simulink model "EcoSIM3_P2_C2_WIP"  (R2014b)
settings: Solver=ode1  SolverMode=SingleTasking  StartTime=0.0  StopTime=inf  FixedStep=0.01  RelTol=1e-3
PostLoadFcn:
  | %, if any(exist('dsrtsu_mdlpostloadfcn', 'file') == [2, 3, 6]), try dsrtsu_mdlpostloadfcn('Execute', bdroot); catch fprintf('Error in PostLoadFcn (dsrtsu_mdlpostloadfcn) for model "%s":\n %s\n', bdroot, lasterr); end, end,
InitFcn:
  | tic
  | %Startup_EcoSIM
values from neighbouring files (symbols this model uses):
  EngPwr = [0 5	10	15	20	25	30	35	40	45	50	55	60	65	70	75	80	85	90	95	100	105	110	115]    [Series_Maps.m]
  EngSpd = [0 477.4645 954.929 1909.858 2864.787 3819.716 4774.645 5729.574 6684.503]    [Series_Maps.m]
  EngTrq = [0	0	0	0	0	0	0	0	0	0	0	0	0	0	0	0	0	0	0	0	0	0	0	0 ... (first row only)    [Series_Maps.m]
  Power = [0 5 10 15 20 25 30]    [Series_Maps.m]
  Torque = [-50,-40,-30,-25,-20,-15,-10,-8,-6,-4,-2,0]    [Series_Maps.m]
undefined symbols (not defined in the file or in its folder): canChannel, Controls, DriveCycles, Driver, EM_EFF_MAP, EM_PwrLoss_MAP, Glbl, Overwritten_Mode, Plants, sigbuilder_block, Trialmap, Veh_Dynamics
libraries: simulink x141, canmsglib x113, fl_lib x104, canlib x89, nesl_utility x56, sdl_lib x29, dspsigops x6, dspswit3 x5, dspstat3 x2, commnoisgen2 x1, dspfdesign x1
(part 4 of 21)

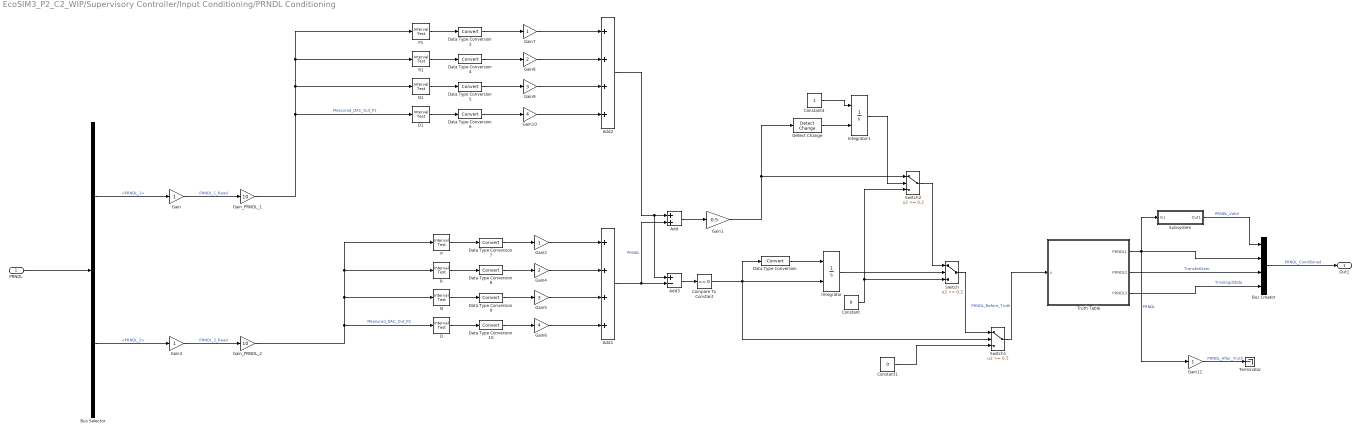
== system EcoSIM3_P2_C2_WIP/Supervisory Controller/Input Conditioning/PRNDL Conditioning ==
  PRNDL : Inport
  Add : Sum
  Add1 : Sum  Inputs=++++
  Add2 : Sum  Inputs=++++
  Add3 : Sum  Inputs=+-
  Bus Creator : BusCreator
  Bus Selector : BusSelector  OutputSignals=GM_Transmit.GM_Electrical_Out.PRNDL_1,GM_Transmit.GM_Electrical_Out.PRNDL_2
  Compare To Constant : simulink/Logic and Bit Operations/Compare To Constant  relop===  const=0  OutDataTypeStr=boolean
  Constant : Constant  Value=0
  Constant1 : Constant  Value=0
  Constant4 : Constant
  D : simulink/Logic and Bit Operations/Interval Test  IntervalClosedRight=on  uplimit=1.90  IntervalClosedLeft=on  lowlimit=1.70  OutDataTypeStr=boolean
  D1 : simulink/Logic and Bit Operations/Interval Test  IntervalClosedRight=on  uplimit=2.2  IntervalClosedLeft=on  lowlimit=1.9  OutDataTypeStr=boolean
  Data Type Conversion{,3..10} (9 alike) : DataTypeConversion
  Detect Change : simulink/Logic and Bit Operations/Detect Change  vinit=0  InputProcessing=Inherited  OutDataTypeStr=boolean
  Gain{,2..3,7,11} (5 alike) : Gain
  Gain1 : Gain  Gain=0.5
  Gain10 : Gain  Gain=4
  Gain4 : Gain  Gain=2
  Gain5 : Gain  Gain=3
  Gain6 : Gain  Gain=4
  Gain8 : Gain  Gain=2
  Gain9 : Gain  Gain=3
  Gain_PRNDL_1 : Gain  Gain=10
  Gain_PRNDL_2 : Gain  Gain=10
  Integrator : Integrator  ExternalReset=either
  Integrator1 : Integrator  ExternalReset=either
  N : simulink/Logic and Bit Operations/Interval Test  IntervalClosedRight=on  uplimit=1.65  IntervalClosedLeft=on  lowlimit=1.35  OutDataTypeStr=boolean
  N1 : simulink/Logic and Bit Operations/Interval Test  IntervalClosedRight=on  uplimit=1.80  IntervalClosedLeft=on  lowlimit=1.55  OutDataTypeStr=boolean
  P : simulink/Logic and Bit Operations/Interval Test  IntervalClosedRight=on  uplimit=0.6  IntervalClosedLeft=on  lowlimit=0.3  OutDataTypeStr=boolean
  P1 : simulink/Logic and Bit Operations/Interval Test  IntervalClosedRight=on  uplimit=0.80  IntervalClosedLeft=on  lowlimit=0.55  OutDataTypeStr=boolean
  R : simulink/Logic and Bit Operations/Interval Test  IntervalClosedRight=on  uplimit=1.25  IntervalClosedLeft=on  lowlimit=1.0  OutDataTypeStr=boolean
  R1 : simulink/Logic and Bit Operations/Interval Test  IntervalClosedRight=on  uplimit=1.45  IntervalClosedLeft=on  lowlimit=1.20  OutDataTypeStr=boolean
  Subsystem : Subsystem
  Switch : Switch  Threshold=0.2
  Switch1 : Switch  Threshold=0.5
  Switch2 : Switch  Threshold=0.2
  Terminator : Terminator
  Truth Table : Truth Table  TreatAsAtomicUnit=on
  Out1 : Outport
  wires:
  Gain_PRNDL_2/1 -> R/1, P/1, N/1, D/1  "Measured_DAC_Out_P2"
  Gain3/1 -> Gain_PRNDL_2/1  "PRNDL_2_Read"
  Bus Selector/2 -> Gain3/1  "<PRNDL_2>"
  Gain_PRNDL_1/1 -> D1/1, N1/1, R1/1, P1/1  "Measured_DAC_Out_P1"
  Gain/1 -> Gain_PRNDL_1/1  "PRNDL_1_Read"
  Bus Selector/1 -> Gain/1  "<PRNDL_1>"
  PRNDL/1 -> Bus Selector/1
  Data Type Conversion7/1 -> Gain2/1
  Data Type Conversion8/1 -> Gain4/1
  Data Type Conversion10/1 -> Gain6/1
  Gain2/1 -> Add1/1
  Gain4/1 -> Add1/2
  Gain5/1 -> Add1/3
  Gain6/1 -> Add1/4
  Data Type Conversion9/1 -> Gain5/1
  Truth Table/1(PRNDL1) -> Bus Creator/2, Subsystem/1(In1), Gain11/1  "PRNDL"
  Truth Table/2(PRNDL2) -> Bus Creator/3  "TransEstGear"
  Truth Table/3(PRNDL3) -> Bus Creator/4  "TrnsEngdState"
  Subsystem/1(Out1) -> Bus Creator/1  "PRNDL_Valid"
  Bus Creator/1 -> Out1/1  "PRNDL_Conditioned"
  P1/1 -> Data Type Conversion3/1
  R1/1 -> Data Type Conversion4/1
  D1/1 -> Data Type Conversion6/1
  Gain7/1 -> Add2/1
  Gain8/1 -> Add2/2
  Gain9/1 -> Add2/3
  Gain10/1 -> Add2/4
  N1/1 -> Data Type Conversion5/1
  Add2/1 -> Add3/1, Add/1
  Add1/1 -> Add/2, Add3/2  "PRNDL"
  Add/1 -> Gain1/1
  Add3/1 -> Compare To Constant/1
  Data Type Conversion/1 -> Integrator/1
  Integrator/1 -> Switch/2
  Constant/1 -> Switch2/3, Switch/3
  Switch1/1 -> Truth Table/1(u)  "PRNDL_Before_Truth"
  Data Type Conversion6/1 -> Gain10/1
  Data Type Conversion5/1 -> Gain9/1
  Data Type Conversion4/1 -> Gain8/1
  Data Type Conversion3/1 -> Gain7/1
  P/1 -> Data Type Conversion7/1
  R/1 -> Data Type Conversion8/1
  D/1 -> Data Type Conversion10/1
  N/1 -> Data Type Conversion9/1
  Compare To Constant/1 -> Integrator/2, Switch1/2, Data Type Conversion/1
  Switch/1 -> Switch1/1
  Constant1/1 -> Switch1/3
  Detect Change/1 -> Integrator1/2
  Constant4/1 -> Integrator1/1
  Integrator1/1 -> Switch2/2
  Gain1/1 -> Detect Change/1, Switch2/1
  Switch2/1 -> Switch/1
  Gain11/1 -> Terminator/1  "PRNDL_After_Truth"

== system EcoSIM3_P2_C2_WIP/Supervisory Controller/Input Conditioning/Velocity Conditioning ==
  Raw Ticks : Inport
  Bus Creator : BusCreator  Inputs=2
  Bus Selector1 : BusSelector  OutputSignals=GM_Transmit.GMLAN_CAN_Out.PPEI_Vehicle_Speed_and_Distance.VehSpdAvgDrvn,GM_Transmit.GMLAN_CAN_Out.PPEI_Driven_Whl_Rotational_Stat.WRSLDWhlDistPlsCntr,GM_Transmit.GMLAN_CAN_Out.PPEI_Driven_Whl_Rotational_Stat.WRSRDWhlDistPlsCntr,GM_Transmit.GMLAN_CAN_Out.PPEI_NonDrivn_Whl_Rotationl_Stat.WRSLNDWhlDistPCntr,GM_Transmit.GMLAN_CAN_Out.PPEI_NonDrivn_Whl_Rotationl_Stat.WRSRNDWhlDistPCntr
  Gain : Gain  Gain=1/3.6
  Mean : dspstat3/Mean  run=off  reset_popup=None  InputProcessing=Columns as channels (frame based)  directionMode=Each column  dimension=1  treatSBRowAsCol=on  roiEnable=off  roiType=Rectangles  roiPortion=Entire ROI  roiOutput=Individual statistics for each ROI  roiFlag=off  outputDataTypeStr=Inherit: Same as accumulator  outputLastDataTypeStr=Inherit: Same as accumulator  outputMin=[]  outputMax=[]  roundingMode=Floor  overflowMode=off
  Mux : Mux
  Subsystem : Subsystem
  Subsystem1 : Subsystem
  Subsystem2 : Subsystem
  Subsystem3 : Subsystem
  Velocity Processed : Outport
  wires:
  Bus Selector1/5 -> Subsystem3/1(In1)  "<WRSRNDWhlDistPCntr>"
  Bus Selector1/4 -> Subsystem2/1(In1)  "<WRSLNDWhlDistPCntr>"
  Raw Ticks/1 -> Bus Selector1/1
  Bus Selector1/1 -> Gain/1  "<VehSpdAvgDrvn>"
  Bus Selector1/3 -> Subsystem1/1(In1)  "<WRSRDWhlDistPlsCntr>"
  Bus Creator/1 -> Velocity Processed/1  "Vehicle_speed"
  Mean/1 -> Bus Creator/2  "Processed_Speed_m_per_sec"
  Gain/1 -> Bus Creator/1  "Vehicle_Speed_meter_per_s"
  Bus Selector1/2 -> Subsystem/1(In1)  "<WRSLDWhlDistPlsCntr>"
  Subsystem2/1(Speed_LND) -> Mux/3
  Subsystem1/1(Speed_RD) -> Mux/2
  Subsystem/1(Speed_LD) -> Mux/1
  Subsystem3/1(Speed_RND) -> Mux/4
  Mux/1 -> Mean/1

== system EcoSIM3_P2_C2_WIP/Supervisory Controller/Mode Operation/Accessory ==
  "Supervisory " : Inport
  CAN : Inport  Port=2
  Enable : EnablePort  StatesWhenEnabling=reset
  BAS_Signals : Subsystem  Commented=on
  BAS_Signals1 : Subsystem
  Bus Creator2 : BusCreator  Inputs=8
  Constant1 : Constant  Value=0
  DC/DC Enabled : Subsystem
  ESS_Messages : Subsystem
  Engine Messages : Subsystem
  Signal Conversion : SignalConversion
  TM Messages : Subsystem
  Trans_Messages : Subsystem
  Output : Outport
  wires:
  Signal Conversion/1 -> Output/1  "HSC_Output"
  Engine Messages/1(Out1) -> Bus Creator2/5
  ESS_Messages/1(Out1) -> Bus Creator2/2  "ESS_Signals_A123"
  Trans_Messages/1(Out1) -> Bus Creator2/6  "Trans_Receive"
  "Supervisory "/1 -> Bus Creator2/7  "Supervisory"
  Bus Creator2/1 -> Signal Conversion/1  "HSC_Output"
  DC/DC Enabled/1(Out1) -> Bus Creator2/8
  TM Messages/1(Out1) -> Bus Creator2/3
  Constant1/1 -> Bus Creator2/1  "Vehicle_Ready"
  CAN/1 -> BAS_Signals1/1(BAS_Speed)
  BAS_Signals1/1(Signals) -> Bus Creator2/4

== system EcoSIM3_P2_C2_WIP/Supervisory Controller/Mode Operation/Charging ==
  From CAN : Inport
  "Supervisory " : Inport  Port=2
  Enable : EnablePort  StatesWhenEnabling=reset
  BAS_Signals : Subsystem  Commented=on
  BAS_Signals1 : Subsystem
  Bus Creator2 : BusCreator  Inputs=8
  Constant2 : Constant  Value=0
  DC/DC Enabled : Subsystem
  EM_Signals : Subsystem
  ESS_Messages : Subsystem
  Engine Messages : Subsystem
  Signal Conversion : SignalConversion
  Trans_Messages : Subsystem
  Output : Outport
  wires:
  Signal Conversion/1 -> Output/1  "HSC_Output"
  Engine Messages/1(Out1) -> Bus Creator2/5
  ESS_Messages/1(Out1) -> Bus Creator2/2  "ESS_Signals_A123"
  Trans_Messages/1(Out1) -> Bus Creator2/6  "Trans_Receive"
  From CAN/1 -> BAS_Signals1/1(BAS_Speed), ESS_Messages/1(From CAN)
  "Supervisory "/1 -> Bus Creator2/7  "Supervisory"
  Bus Creator2/1 -> Signal Conversion/1  "HSC_Output"
  EM_Signals/1(Out1) -> Bus Creator2/3
  DC/DC Enabled/1(Out1) -> Bus Creator2/8
  Constant2/1 -> Bus Creator2/1  "Vehicle_Ready"
  BAS_Signals1/1(Signals) -> Bus Creator2/4

== system EcoSIM3_P2_C2_WIP/Supervisory Controller/Mode Operation/EV ==
  "Supervisory " : Inport
  CAN : Inport  Port=2
  Enable : EnablePort  StatesWhenEnabling=reset
  BAS_Signals : Subsystem  Commented=on
  BAS_Signals1 : Subsystem
  Bus Creator1 : BusCreator  Inputs=8
  Bus Creator2 : BusCreator  Inputs=3
  Bus Selector : BusSelector  OutputSignals=Driver Torque Request
  Bus Selector1 : BusSelector  OutputSignals=EM_Transmit.EM_CAN_Out.M165_Motor_Position_Info.Motor_Speed,EM_Transmit.EM_CAN_Out.M162_Temperature_Set_3.Motor_Temperature
  Constant1 : Constant  Value=0
  Constant2 : Constant
  Constant4 : Constant
  Constant5 : Constant  Value=0
  DC/DC Enabled : Subsystem
  EM Max Torque1 : Lookup_n-D  NumberOfTableDimensions=1  BreakpointsForDimension1=Plants.EM.Mdl.Plant.max_min_RPM  BreakpointsForDimension2=[25,70]  Table=[Plants.EM.Mdl.Plant.T_max_Peak]  InternalRulePriority=Speed  RndMeth=Simplest  InputSameDT=on
  ESS_Messages : Subsystem
  Engine Messages : Subsystem
  Gain : Gain  Gain=1/(2.77*2.77)
  Saturation Dynamic : simulink/Discontinuities/Saturation Dynamic  OutMin=[]  OutMax=[]  OutDataTypeStr=Inherit: Same as second input  OutDataType=fixdt(1, 16)  OutScaling=2^-10  DoSatur=off
  Scope : Scope
      settings: SaveName=ScopeData67
  Signal Conversion : SignalConversion
  Trans_Messages : Subsystem
  Output : Outport
  wires:
  Signal Conversion/1 -> Output/1  "HSC_Output"
  Engine Messages/1(Out1) -> Bus Creator1/5
  ESS_Messages/1(Out1) -> Bus Creator1/2  "ESS_Signals_A123"
  Bus Creator2/1 -> Bus Creator1/3  "EM_Messages_Rhinehart"
  Gain/1 -> Saturation Dynamic/2  "Torque_Command"
  Constant1/1 -> Bus Creator2/3  "Rotation_Direction"
  Constant2/1 -> Bus Creator2/1  "Inverter_Enable"
  Trans_Messages/1(Out1) -> Bus Creator1/6  "Trans_Receive"
  "Supervisory "/1 -> Bus Creator1/7, Bus Selector/1  "Supervisory"
  Bus Creator1/1 -> Signal Conversion/1  "HSC_Output"
  Bus Selector/1 -> Gain/1  "<Driver Torque Request>"
  Constant4/1 -> Bus Creator1/1  "Vehicle_Ready"
  DC/DC Enabled/1(Out1) -> Bus Creator1/8
  Saturation Dynamic/1 -> Bus Creator2/2  "Torque_Command"
  Constant5/1 -> Saturation Dynamic/3
  CAN/1 -> BAS_Signals1/1(BAS_Speed), Bus Selector1/1
  Bus Selector1/1 -> EM Max Torque1/1  "<Motor_Speed>"
  Bus Selector1/2 -> ?  "<Motor_Temperature>"
  EM Max Torque1/1 -> Scope/1, Saturation Dynamic/1
  BAS_Signals1/1(Signals) -> Bus Creator1/4

== system EcoSIM3_P2_C2_WIP/Supervisory Controller/Mode Operation/Engine Only  ==
  note: this will end up being engine idle in the vehicle
  "Supervisory " : Inport
  From CAN : Inport  Port=2
  Enable : EnablePort  StatesWhenEnabling=reset
  BAS_Signals : Subsystem  Commented=on
  BAS_Signals1 : Subsystem
  Bus Creator1 : BusCreator  Inputs=8
  Bus Creator6 : BusCreator  Commented=on  Inputs=2
  Constant1 : Constant  Commented=on
  Constant2 : Constant  Commented=on  Value=0
  Constant4 : Constant
  DC/DC Enabled : Subsystem
  ESS_Messages : Subsystem
  Engine Messages : Subsystem  Commented=on
  Engine Messages1 : Subsystem
  "ICE Torque Request & Gear Selection " : Subsystem
  Signal Conversion : SignalConversion
  Subsystem : Subsystem  Commented=on
  Supervisory 1 : InportShadow
  TM Messages : Subsystem
  Terminator : Terminator  Commented=on
  Terminator1 : Terminator  Commented=on
  Trans Clutch Messages : Subsystem
  "Output " : Outport
  wires:
  Signal Conversion/1 -> "Output "/1  "HSC_Output"
  ESS_Messages/1(Out1) -> Bus Creator1/2  "ESS_Signals_A123"
  BAS_Signals1/1(Signals) -> Bus Creator1/4
  Subsystem/3("Gear Requested ") -> Terminator1/1  "Gear_Request"
  "Supervisory "/1 -> Bus Creator1/7  "Supervisory"
  Bus Creator1/1 -> Signal Conversion/1  "HSC_Output"
  Subsystem/2(Shift Requested) -> Terminator/1
  Constant4/1 -> Bus Creator1/1  "Vehicle_Ready"
  DC/DC Enabled/1(Out1) -> Bus Creator1/8
  TM Messages/1(Out1) -> Bus Creator1/3  "EM_Messages_Rhinehart"
  Engine Messages1/1(Out1) -> Bus Creator1/5
  Supervisory 1/1 -> TM Messages/1(Supervisory)  "Supervisory"
  From CAN/1 -> "ICE Torque Request & Gear Selection "/1(CAN), Trans Clutch Messages/2(CAN), TM Messages/2(CAN), BAS_Signals1/1(BAS_Speed)
  "ICE Torque Request & Gear Selection "/1(ICE_Torque_Request [Nm]) -> Engine Messages1/1(Torque)
  "ICE Torque Request & Gear Selection "/2(Gear_Request[-]) -> Trans Clutch Messages/1(Gear Request)
  Trans Clutch Messages/1(Out1) -> Bus Creator1/6
  Constant2/1 -> Bus Creator6/1  "Shift_Request"
  Constant1/1 -> Bus Creator6/2  "Gear_Request"

== system EcoSIM3_P2_C2_WIP/Supervisory Controller/Mode Operation/Engine Start  ==
  "Supervisory " : Inport
  "CAN In " : Inport  Port=2
  Enable : EnablePort  StatesWhenEnabling=reset
  1-D Lookup Table : Lookup_n-D  NumberOfTableDimensions=1  BreakpointsForDimension1=[0 2699 2700 3000 3239 3240]  Table=[11.11 11.11 8 5.5 5.5 0]  InternalRulePriority=Speed  RndMeth=Simplest  InputSameDT=on
  BAS_Signals1 : Subsystem
  Bus Creator1 : BusCreator  Inputs=8
  Bus Creator2 : BusCreator  Inputs=3
  Bus Creator4 : BusCreator  Inputs=3
  Bus Selector : BusSelector  OutputSignals=BAS_Transmit.BAS_CAN_Out.Status_1.BAS_Speed_rad_per_s
  Compare To Constant : simulink/Logic and Bit Operations/Compare To Constant  relop=>  const=900  OutDataTypeStr=boolean
  Constant1 : Constant  Value=0
  Constant3 : Constant  Value=0
  Constant4 : Constant
  Constant5 : Constant
  Constant6 : Constant
  Convert to Engine Speed : Gain  Gain=1/2.7
  DC/DC Enabled : Subsystem
  Data Type Conversion : DataTypeConversion  OutDataTypeStr=double
  ESS_Messages : Subsystem
  Engine Messages : Subsystem
  Sample and Hold : dspsigops/Sample and Hold  trig=Rising edge  initCond=0  latchinput=off
  Signal Conversion : SignalConversion
  Supervisory 1 : InportShadow
  TM Messages : Subsystem
  Trans Messages : Subsystem
  rad/sec to RPM : Gain  Gain=9.54929659643
  rad/sec to RPM1 : Gain  Gain=1.1
  "Output " : Outport
  wires:
  Signal Conversion/1 -> "Output "/1  "HSC_Output"
  ESS_Messages/1(Out1) -> Bus Creator1/2  "ESS_Signals_A123"
  "Supervisory "/1 -> Bus Creator1/7  "Supervisory"
  Bus Creator1/1 -> Signal Conversion/1  "HSC_Output"
  Constant5/1 -> Bus Creator1/1  "Vehicle_Ready"
  DC/DC Enabled/1(Out1) -> Bus Creator1/8
  TM Messages/1(Out1) -> Bus Creator1/3
  Constant6/1 -> Bus Creator4/3  "BAS_Mode_Request"
  Trans Messages/1(Out1) -> Bus Creator1/6
  Supervisory 1/1 -> TM Messages/1(In1)  "Supervisory"
  Constant3/1 -> Bus Creator2/1  "ICE_Torque_Request_Nm"
  1-D Lookup Table/1 -> rad/sec to RPM1/1  "BAS_Torque_Request_Nm"
  Constant1/1 -> Bus Creator4/2  "BAS_Speed_Request"
  Constant4/1 -> Bus Creator2/2  "Engine_On"
  "CAN In "/1 -> BAS_Signals1/1(BAS_Speed), Bus Selector/1
  Bus Selector/1 -> Engine Messages/1(In1), rad/sec to RPM/1  "<BAS_Speed_rad_per_s>"
  rad/sec to RPM/1 -> 1-D Lookup Table/1, Convert to Engine Speed/1  "BAS_Speed_RPM"
  Compare To Constant/1 -> Data Type Conversion/1
  Convert to Engine Speed/1 -> Compare To Constant/1
  Data Type Conversion/1 -> Sample and Hold/Trigger, Sample and Hold/1  "Engine_Run"
  Sample and Hold/1 -> Bus Creator2/3  "Engine_Run"
  rad/sec to RPM1/1 -> Bus Creator4/1  "BAS_Torque_Request_Nm"
  BAS_Signals1/1(Signals) -> Bus Creator1/4
  Engine Messages/1(Out1) -> Bus Creator1/5

== system EcoSIM3_P2_C2_WIP/Supervisory Controller/Mode Operation/Limited EV ==
  "Supervisory " : Inport
  CAN : Inport  Port=2
  Enable : EnablePort  StatesWhenEnabling=reset
  BAS_Signals : Subsystem  Commented=on
  BAS_Signals1 : Subsystem
  Bus Creator3 : BusCreator  Inputs=8
  Bus Creator4 : BusCreator  Inputs=3
  Bus Selector : BusSelector  OutputSignals=Driver Torque Request
  Bus Selector1 : BusSelector  OutputSignals=ESS_Transmit.ESS_CAN_Out.BCM_Limits.bcm_dis_buf,EM_Transmit.EM_CAN_Out.M162_Temperature_Set_3.Motor_Temperature,EM_Transmit
  Constant1 : Constant
  Constant2 : Constant  Value=0
  Constant4 : Constant
  DC/DC Enabled : Subsystem
  ESS_Messages : Subsystem
  Gain1 : Gain  Gain=1/(2.77*2.77)
  ICE_torque : Subsystem
  "Inverter Temp Selection " : Subsystem
  Signal Conversion : SignalConversion
  Subsystem : Subsystem
  Temperature Limiting Disbuf : Subsystem
  Temperature Limiting Old : Subsystem  Commented=on
  Output : Outport
  wires:
  Signal Conversion/1 -> Output/1  "HSC_Output"
  ESS_Messages/1(Out1) -> Bus Creator3/2  "ESS_Signals_A123"
  Bus Creator4/1 -> Bus Creator3/3  "EM_Messages_Rhinehart"
  Bus Selector/1 -> Subsystem/1(Driver_request), Gain1/1  "<Driver Torque Request>"
  Constant2/1 -> Bus Creator4/3  "Rotation_Direction"
  Constant4/1 -> Bus Creator4/1  "Inverter_Enable"
  "Supervisory "/1 -> Bus Creator3/7, Bus Selector/1  "Supervisory"
  Bus Creator3/1 -> Signal Conversion/1  "HSC_Output"
  Constant1/1 -> Bus Creator3/1  "Vehicle_Ready"
  DC/DC Enabled/1(Out1) -> Bus Creator3/8
  Gain1/1 -> Temperature Limiting Disbuf/2(Torque Request)  "Torque_Command"
  "Inverter Temp Selection "/1(Out1) -> Temperature Limiting Disbuf/5("Inverter Temperature ")
  CAN/1 -> ICE_torque/2(CAN), BAS_Signals1/1(BAS_Speed), Bus Selector1/1
  Temperature Limiting Disbuf/1(EM_torque Command) -> Bus Creator4/2  "Torque_Command"
  Bus Selector1/3 -> "Inverter Temp Selection "/1(In1)  "<EM_Transmit>"
  BAS_Signals1/1(Signals) -> Bus Creator3/4
  Subsystem/1(EM_trq) -> [EM_trq]
  Subsystem/2(ICE_trq) -> [ICE_trq_req]
  [EM_trq] -> Temperature Limiting Disbuf/1(ESS_trq_limit)
  Bus Selector1/2 -> Temperature Limiting Disbuf/4("Motor Temperature ")  "<Motor_Temperature>"
  Bus Selector1/1 -> Subsystem/2(ESS discharge buffer), Temperature Limiting Disbuf/3(ESS discharge buffer)  "<bcm_dis_buf>"
  ICE_torque/2(Trans_Receive) -> Bus Creator3/6
  ICE_torque/1(ICE_Request) -> Bus Creator3/5
  [ICE_trq_req] -> ICE_torque/1(ICE_torque_request)

== system EcoSIM3_P2_C2_WIP/Supervisory Controller/Mode Operation/Series ==
  "Supervisory " : Inport
  From CAN : Inport  Port=2
  Enable : EnablePort  StatesWhenEnabling=reset
  Bus Creator1 : BusCreator  Inputs=8
  Bus Creator2 : BusCreator  Inputs=3
  Bus Creator4 : BusCreator  Inputs=3
  Bus Creator5 : BusCreator  Inputs=3
  Bus Selector : BusSelector  OutputSignals=Driver Torque Request
  Constant1 : Constant  Value=2
  Constant{2,5,7..8} (4 alike) : Constant
  Constant3 : Constant  Value=0
  Constant4 : Constant  Value=0
  DC/DC Enabled : Subsystem
  ESS_Messages : Subsystem
  Gain : Gain
  Gain1 : Gain  Gain=1/(2.77*2.77)
  "Series Torque Determination " : Subsystem
  Signal Conversion : SignalConversion
  Supervisory 1 : InportShadow
  Trans_Messages : Subsystem
  "Output " : Outport
  wires:
  Bus Creator1/1 -> Signal Conversion/1  "HSC_Output"
  "Supervisory "/1 -> Bus Creator1/7  "Supervisory"
  Bus Selector/1 -> Gain1/1  "<Driver Torque Request>"
  Supervisory 1/1 -> Bus Selector/1  "Supervisory"
  Constant5/1 -> Bus Creator5/1  "Inverter_Enable"
  Constant3/1 -> Bus Creator5/3  "Rotation_Direction"
  Bus Creator5/1 -> Bus Creator1/3  "EM_Messages_Rhinehart"
  ESS_Messages/1(Out1) -> Bus Creator1/2  "ESS_Signals_A123"
  Signal Conversion/1 -> "Output "/1  "HSC_Output"
  Trans_Messages/1(Out1) -> Bus Creator1/6  "Trans_Receive"
  Bus Creator4/1 -> Bus Creator1/4  "BAS_SoftECU_Receive"
  Constant1/1 -> Bus Creator4/3  "BAS_Mode_Request"
  DC/DC Enabled/1(Out1) -> Bus Creator1/8
  Constant2/1 -> Bus Creator1/1  "Vehicle_Ready"
  Gain1/1 -> Bus Creator5/2  "Torque_Command"
  "Series Torque Determination "/2(Engine Torque) -> Gain/1
  "Series Torque Determination "/1(BAS Speed) -> Bus Creator4/2  "BAS_Speed_Request"
  Constant4/1 -> Bus Creator4/1  "BAS_Torque_Request_Nm"
  From CAN/1 -> "Series Torque Determination "/1(Battery SOC)
  Gain/1 -> Bus Creator2/1  "ICE_Torque_Request_Nm"
  Constant7/1 -> Bus Creator2/2  "Engine_On"
  Constant8/1 -> Bus Creator2/3  "Engine_Run"
  Bus Creator2/1 -> Bus Creator1/5  "ICE_Request"

== system EcoSIM3_P2_C2_WIP/Supervisory Controller/Mode Operation/Series1 ==
  From CAN : Inport
  "Supervisory " : Inport  Port=2
  Enable : EnablePort  StatesWhenEnabling=reset
  BAS_Signals : Subsystem
  Bus Creator1 : BusCreator  Inputs=8
  Bus Creator2 : BusCreator  Inputs=3
  Bus Selector : BusSelector  OutputSignals=BAS_Transmit.BAS_CAN_Out.Status_1.BAS_Speed_rad_per_s
  Bus Selector1 : BusSelector  OutputSignals=EM_Transmit.EM_CAN_Out.M165_Motor_Position_Info.Motor_Speed
  Bus Selector2 : BusSelector  OutputSignals=Driver Torque Request
  Constant1 : Constant  Value=410
  Constant2 : Constant
  Constant3 : Constant  Value=0
  Constant4 : Constant
  Constant5 : Constant  Value=0
  DC/DC Enabled : Subsystem
  EM Max Torque1 : Lookup_n-D  NumberOfTableDimensions=1  BreakpointsForDimension1=Plants.EM.Mdl.Plant.max_min_RPM  BreakpointsForDimension2=[25,70]  Table=[Plants.EM.Mdl.Plant.T_max_Peak]  InternalRulePriority=Speed  RndMeth=Simplest  InputSameDT=on
  ESS_Messages : Subsystem
  Engine Messages : Subsystem
  Engine Torque Request : Stateflow chart  TreatAsAtomicUnit=on
  Engine Torque Request1 : Stateflow chart  Commented=on  TreatAsAtomicUnit=on
  Gain : Gain  Gain=1/(2.77*2.77)
  Saturation Dynamic : simulink/Discontinuities/Saturation Dynamic  OutMin=[]  OutMax=[]  OutDataTypeStr=Inherit: Same as second input  OutDataType=fixdt(1, 16)  OutScaling=2^-10  DoSatur=off
  Signal Conversion : SignalConversion
  Supervisory 1 : InportShadow  Port=2
  Trans_Messages : Subsystem
  "Output " : Outport
  wires:
  BAS_Signals/1(Signals) -> Bus Creator1/4
  Engine Messages/1(Out1) -> Bus Creator1/5
  DC/DC Enabled/1(Out1) -> Bus Creator1/8
  Constant4/1 -> Bus Creator1/1  "Vehicle_Ready"
  From CAN/1 -> Bus Selector1/1, Bus Selector/1, BAS_Signals/1(BAS_Speed)
  Bus Creator1/1 -> Signal Conversion/1  "HSC_Output"
  "Supervisory "/1 -> Bus Creator1/7  "Supervisory"
  Signal Conversion/1 -> "Output "/1  "HSC_Output"
  Bus Selector/1 -> Engine Torque Request/1(BAS_Speed)  "<BAS_Speed_rad_per_s>"
  Engine Torque Request/1(Torque_Request) -> Engine Messages/1(Engine_Torque_Request)  "ICE_Torque_Request_Nm"
  Constant1/1 -> Engine Torque Request/2(Desired_BAS_Speed), BAS_Signals/2(Desired_BAS_Speed)
  ESS_Messages/1(Out1) -> Bus Creator1/2  "ESS_Signals_A123"
  Bus Creator2/1 -> Bus Creator1/3  "EM_Messages_Rhinehart"
  Gain/1 -> Saturation Dynamic/2  "Torque_Command"
  Constant3/1 -> Bus Creator2/3  "Rotation_Direction"
  Constant2/1 -> Bus Creator2/1  "Inverter_Enable"
  Bus Selector2/1 -> Gain/1  "<Driver Torque Request>"
  Saturation Dynamic/1 -> Bus Creator2/2  "Torque_Command"
  Constant5/1 -> Saturation Dynamic/3
  Bus Selector1/1 -> EM Max Torque1/1  "<Motor_Speed>"
  EM Max Torque1/1 -> Saturation Dynamic/1
  Supervisory 1/1 -> Bus Selector2/1  "Supervisory"
  Trans_Messages/1(Out1) -> Bus Creator1/6  "Trans_Receive"

== system EcoSIM3_P2_C2_WIP/Supervisory Controller/Mode Operation/Shutdown ==
  From CAN : Inport
  "Supervisory " : Inport  Port=2
  Enable : EnablePort  StatesWhenEnabling=reset
  BAS_Signals : Subsystem  Commented=on
  BAS_Signals1 : Subsystem
  Bus Creator2 : BusCreator  Inputs=8
  Bus Creator3 : BusCreator  Inputs=3
  Constant1 : Constant  Value=0
  Constant3 : Constant  Value=0
  Constant6 : Constant  Value=0
  DC/DC Disabled : Subsystem
  Engine Messages : Subsystem
  Shutdown : Subsystem
  Shutdown Complete : Subsystem
  Signal Conversion : SignalConversion
  Trans_Messages : Subsystem
  Output : Outport
  wires:
  Signal Conversion/1 -> Output/1  "HSC_Output"
  Engine Messages/1(Out1) -> Bus Creator2/5
  Shutdown/1(Out1) -> Shutdown Complete/1(In1), Bus Creator2/2
  Bus Creator3/1 -> Bus Creator2/3  "EM_Messages_Rhinehart"
  Constant6/1 -> Bus Creator3/2  "Torque_Command"
  Constant3/1 -> Bus Creator3/3  "Rotation_Direction"
  Constant1/1 -> Shutdown Complete/2(In2), Bus Creator3/1  "Inverter_Enable"
  Trans_Messages/1(Out1) -> Bus Creator2/6  "Trans_Receive"
  From CAN/1 -> BAS_Signals1/1(BAS_Speed), Shutdown/1(In1)
  "Supervisory "/1 -> Bus Creator2/7  "Supervisory"
  Bus Creator2/1 -> Signal Conversion/1  "HSC_Output"
  DC/DC Disabled/1(Out1) -> Bus Creator2/8
  Shutdown Complete/1(Out1) -> Bus Creator2/1  "Vehicle_Ready"
  BAS_Signals1/1(Signals) -> Bus Creator2/4

== system EcoSIM3_P2_C2_WIP/Supervisory Controller/Mode Operation/Startup ==
  From CAN : Inport
  "Supervisory " : Inport  Port=2
  Enable : EnablePort  StatesWhenEnabling=reset
  BAS Start up : Subsystem
  BAS_Signals : Subsystem
  "Battery Start Up " : Subsystem
  Bus Creator1 : BusCreator  Inputs=8
  Bus Selector : BusSelector  OutputSignals=ESS_Transmit.ESS_CAN_Out.BCM_Status.bcm_mainc_stat
  Bus Selector1 : BusSelector  OutputSignals=Inverter_Enable
  Bus Selector2 : BusSelector  OutputSignals=ModeReq
  DC/DC Enabled : Subsystem
  EM Start up : Subsystem
  Engine Messages : Subsystem
  Signal Conversion : SignalConversion
  "Start up overide " : Subsystem
  To Workspace : ToWorkspace  VariableName=StartComplete  SaveFormat=Structure With Time  SampleTime=-1
  To Workspace1 : ToWorkspace  VariableName=bcm_mainc_stat  SaveFormat=Structure With Time  SampleTime=-1
  To Workspace2 : ToWorkspace  VariableName=Inverter_enable  SaveFormat=Structure With Time  SampleTime=-1
  To Workspace3 : ToWorkspace  VariableName=BAS_Enabled  SaveFormat=Structure With Time  SampleTime=-1
  To Workspace4 : ToWorkspace  VariableName=VehReady2  SaveFormat=Structure With Time  SampleTime=-1
  Trans_Messages : Subsystem
  Vehicle Ready : Stateflow chart  TreatAsAtomicUnit=on
  "Vehicle Start Up " : Subsystem
  Output : Outport
  wires:
  Bus Creator1/1 -> Signal Conversion/1
  Trans_Messages/1(Out1) -> Bus Creator1/6  "Trans_Receive"
  "Battery Start Up "/1(Out1) -> Bus Creator1/2
  EM Start up/1(Out1) -> Bus Selector1/1, Bus Creator1/3
  Bus Selector/1 -> To Workspace1/1, Vehicle Ready/2(bcm_mainc_stat)  "<bcm_mainc_stat>"
  Bus Selector1/1 -> Vehicle Ready/3(Inverter_Enable), To Workspace2/1  "<Inverter_Enable>"
  Bus Selector2/1 -> To Workspace3/1, Vehicle Ready/4(BAS_Mode_Request)  "<ModeReq>"
  Vehicle Ready/1(Vehicle_Ready) -> To Workspace4/1, Bus Creator1/1  "Vehicle_Ready"
  "Supervisory "/1 -> Bus Creator1/7  "Supervisory"
  Signal Conversion/1 -> Output/1  "HSC_Output"
  "Vehicle Start Up "/1(Start) -> Vehicle Ready/1(Startup_Complete), To Workspace/1
  From CAN/1 -> "Start up overide "/1(In1), BAS_Signals/1(BAS_Speed), BAS Start up/1(In1), EM Start up/1(In1), "Battery Start Up "/1(CAN), Bus Selector/1
  DC/DC Enabled/1(Out1) -> Bus Creator1/8
  Engine Messages/1(Out1) -> Bus Creator1/5
  "Start up overide "/1(Out1) -> "Vehicle Start Up "/1(In1)
  BAS_Signals/1(Signals) -> Bus Creator1/4, Bus Selector2/1

== system EcoSIM3_P2_C2_WIP/Supervisory Controller/Mode Selection /Limp Home Mode Selection   ==
  "Mode Requested  " : Inport
  "Fault Code " : Inport  Port=2
  Chart : Stateflow chart  TreatAsAtomicUnit=on
  Data Type Conversion : DataTypeConversion  OutDataTypeStr=double
  Fault Counter : Subsystem
  Sample and Hold : dspsigops/Sample and Hold  trig=Rising edge  initCond=0  latchinput=off
  Scope : Scope
      settings: YMin=1.625  YMax=5.375  SaveName=ScopeData6
  Switch : Switch  Criteria=u2 > Threshold  OutDataTypeStr=Inherit: Inherit via back propagation
  Transport Delay : TransportDelay  DelayTime=.1
  Vehicle Mode : Outport
  wires:
  "Mode Requested  "/1 -> Switch/3
  Switch/1 -> Vehicle Mode/1
  Chart/1(VEH_Mode) -> Scope/1, Switch/1
  "Fault Code "/1 -> Data Type Conversion/1
  Fault Counter/1(Fault_Code) -> Chart/1(Fault_Code)
  Sample and Hold/1 -> Switch/2
  Transport Delay/1 -> Fault Counter/1(In1), Sample and Hold/1, Sample and Hold/Trigger
  Data Type Conversion/1 -> Transport Delay/1

== system EcoSIM3_P2_C2_WIP/Supervisory Controller/Mode Selection /Start-Stop control ==
  From_CAN : Inport
  Startup : Inport  Port=2
  Bus Selector : BusSelector  OutputSignals=Vehicle_speed.Vehicle_Speed_meter_per_s,GM_Transmit.GMLAN_CAN_Out.PPEI_Brake_Apply_Status.BrkPdlPos,Alpha_percent
  Bus Selector1 : BusSelector  OutputSignals=ICE_Request.Engine_On,ICE_Request.Engine_Run
  Bus Selector2 : BusSelector  OutputSignals=Vehicle_speed.Vehicle_Speed_meter_per_s,GM_Transmit.GMLAN_CAN_Out.PPEI_Brake_Apply_Status.BrkPdlPos
  Compare To Constant : simulink/Logic and Bit Operations/Compare To Constant  relop===  const=4.0  OutDataTypeStr=boolean
  Compare To Constant1 : simulink/Logic and Bit Operations/Compare To Constant  relop=>  const=1  OutDataTypeStr=boolean
  Compare To Constant2 : simulink/Logic and Bit Operations/Compare To Constant  relop=<=  const=2  OutDataTypeStr=boolean
  Compare To Constant3 : simulink/Logic and Bit Operations/Compare To Constant  relop===  const=2  OutDataTypeStr=boolean
  Compare To Constant4 : simulink/Logic and Bit Operations/Compare To Constant  relop===  const=3.0  OutDataTypeStr=boolean
  Constant : Constant  Value=3
  Constant1 : Constant  Value=Plants.ICE.Mdl.Plant.clutch_w
  Constant2 : Constant  Value=9
  Constant3 : Constant  Commented=on  Value=Overwritten_Mode
  Constant4 : Constant  Value=3
  Constant5 : Constant  Value=2
  Constant6 : Constant  Value=2
  Constant7 : Constant
  Data Type Conversion : DataTypeConversion
  Engine_Start_Stop : Stateflow chart  TreatAsAtomicUnit=on
  From_CAN1 : InportShadow
  Integrator : Integrator  ExternalReset=rising
  Logical Operator : Logic  AllPortsSameDT=off  OutDataTypeStr=boolean
  Logical Operator1 : Logic  AllPortsSameDT=off  OutDataTypeStr=boolean
  Memory1 : Memory
  Memory2 : Memory
  Mode Overide1 : Switch  Criteria=u2 > Threshold  Threshold=0.5
  Multiport Switch : MultiPortSwitch
  Terminator : Terminator
  Terminator1 : Terminator
  Terminator2 : Terminator
  Mode : Outport
  wires:
  Compare To Constant1/1 -> Logical Operator1/2
  Logical Operator1/1 -> Mode Overide1/2
  Compare To Constant2/1 -> Logical Operator1/1
  Constant2/1 -> Mode Overide1/1
  Constant/1 -> Mode Overide1/3
  From_CAN/1 -> Bus Selector/1
  Startup/1 -> Bus Selector1/1
  Bus Selector1/1 -> Memory1/1  "<Engine_On>"
  Bus Selector1/2 -> Memory2/1  "<Engine_Run>"
  Engine_Start_Stop/1(Mode) -> Multiport Switch/3
  Mode Overide1/1 -> Multiport Switch/4
  Constant5/1 -> Multiport Switch/1
  Constant4/1 -> Multiport Switch/2
  Multiport Switch/1 -> Compare To Constant3/1, Compare To Constant4/1, Compare To Constant/1, Mode/1
  Engine_Start_Stop/2(Time_in_wait) -> Integrator/2, Integrator/1
  Compare To Constant3/1 -> Terminator2/1  "Engine_Stop"
  Compare To Constant4/1 -> Terminator1/1  "Engine_Only"
  Compare To Constant/1 -> Terminator/1  "Engine_Start"
  Bus Selector/1 -> Engine_Start_Stop/1(Vehicle_Speed)  "<Vehicle_Speed_meter_per_s>"
  Bus Selector/2 -> Engine_Start_Stop/2(Brake_Pedal_Position)  "<BrkPdlPos>"
  Bus Selector/3 -> Engine_Start_Stop/3(Alpha_Percent)  "<Alpha_percent>"
  Memory1/1 -> Logical Operator/1
  Memory2/1 -> Logical Operator/2
  Constant7/1 -> Engine_Start_Stop/4(eng_running)
  Logical Operator/1 -> Data Type Conversion/1
  Integrator/1 -> Engine_Start_Stop/6(Time_to_Stop)
  Constant6/1 -> Engine_Start_Stop/5(Time_in_wait_limit)
  From_CAN1/1 -> Bus Selector2/1
  Bus Selector2/1 -> Compare To Constant2/1  "<Vehicle_Speed_meter_per_s>"
  Bus Selector2/2 -> Compare To Constant1/1  "<BrkPdlPos>"

== system EcoSIM3_P2_C2_WIP/Supervisory Controller/PRNDL/Determine Gear ==
  From CAN : Inport
  HSC Inputs : Inport  Port=2
  Bus Selector : BusSelector  OutputSignals=GM_Transmit.GM_Electrical_Out.PRNDL,ESS_Transmit.ESS_CAN_Out.BCM_Status.bcm_epo,GM_Transmit.GMLAN_CAN_Out.PPEI_Platform_General_Status.SysPwrMd,ESS_Transmit.ESS_CAN_Out.BCM_Status.bcm_on_plug
  Bus Selector1 : BusSelector  OutputSignals=Vehicle_Ready
  Compare To Constant : simulink/Logic and Bit Operations/Compare To Constant  relop=<  const=2  OutDataTypeStr=boolean  ZeroCross=off
  Data Type Conversion : DataTypeConversion
  Display{,1..5} (6 alike) : Display
  Logical Operator : Logic  Operator=OR  Inputs=4  AllPortsSameDT=off  OutDataTypeStr=boolean
  Logical Operator1 : Logic  Operator=NOT  AllPortsSameDT=off  OutDataTypeStr=boolean
  Subsystem : Subsystem
  Truth Table : Truth Table  TreatAsAtomicUnit=on
  Gear : Outport
  wires:
  Bus Selector/1 -> Display/1, Subsystem/1(PRNDL Position), Truth Table/1(PRNDL)  "<PRNDL>"
  From CAN/1 -> Bus Selector/1
  Logical Operator/1 -> Truth Table/3(Force_Park)
  Logical Operator1/1 -> Data Type Conversion/1
  Data Type Conversion/1 -> Logical Operator/4
  Compare To Constant/1 -> Logical Operator/2
  Bus Selector/4 -> Logical Operator/3, Display3/1  "<bcm_on_plug>"
  Bus Selector1/1 -> Display4/1, Logical Operator1/1  "<Vehicle_Ready>"
  Truth Table/1(y) -> Display5/1, Gear/1
  Bus Selector/3 -> Display2/1, Compare To Constant/1  "<SysPwrMd>"
  HSC Inputs/1 -> Bus Selector1/1
  Bus Selector/2 -> Display1/1, Subsystem/2(bcm_epo)  "<bcm_epo>"
  Subsystem/1(Force Neutral) -> Truth Table/2(Force_Neutral)
  Subsystem/2(Force Park) -> Logical Operator/1

== system EcoSIM3_P2_C2_WIP/Supervisory Controller/PRNDL/Determine Gear1 ==
  In1 : Inport
  In2 : Inport  Port=2
  Bus Selector : BusSelector  OutputSignals=GM_Transmit.GM_Electrical_Out.PRNDL,ESS_Transmit.ESS_CAN_Out.BCM_Status.bcm_epo,GM_Transmit.GM_Electrical_Out.Key_State
  Bus Selector1 : BusSelector  OutputSignals=Vehicle_Ready
  Compare To Constant : simulink/Logic and Bit Operations/Compare To Constant  relop=<  const=2  OutDataTypeStr=boolean  ZeroCross=off
  Data Type Conversion : DataTypeConversion
  Logical Operator : Logic  Operator=OR  Inputs=4  AllPortsSameDT=off  OutDataTypeStr=boolean
  Logical Operator1 : Logic  Operator=NOT  AllPortsSameDT=off  OutDataTypeStr=boolean
  Truth Table : Truth Table  TreatAsAtomicUnit=on
  bcm_on_plug : Constant  Value=0
  Gear : Outport
  wires:
  Bus Selector/1 -> Truth Table/1(PRNDL)  "<PRNDL>"
  In1/1 -> Bus Selector/1
  Truth Table/1(y) -> Gear/1
  Logical Operator/1 -> Truth Table/2(Force_Neutral)
  Bus Selector/3 -> Compare To Constant/1  "<Key_State>"
  In2/1 -> Bus Selector1/1
  Logical Operator1/1 -> Data Type Conversion/1
  Data Type Conversion/1 -> Logical Operator/3
  Compare To Constant/1 -> Logical Operator/4
  bcm_on_plug/1 -> Logical Operator/1
  Bus Selector/2 -> Logical Operator/2  "<bcm_epo>"
  Bus Selector1/1 -> Logical Operator1/1  "<Vehicle_Ready>"

== system EcoSIM3_P2_C2_WIP/Supervisory Controller/PRNDL/Drive ==
  In1 : Inport
  CAN : Inport  Port=2
  Clutch : Inport  Port=3
  Enable : EnablePort
  Bus Creator : BusCreator  Inputs=6
  Bus Creator1 : BusCreator  Inputs=3
  Bus Creator4 : BusCreator  Inputs=3
  Bus Selector : BusSelector  OutputSignals=ESS_Signals_A123,EM_Messages_Rhinehart.Inverter_Enable,EM_Messages_Rhinehart.Torque_Command,EM_Messages_Rhinehart.Rotation_Direction,BAS_Infineon_Messages,ICE_Request.ICE_Torque_Request_Nm,ICE_Request.Engine_On,ICE_Request.Engine_Run,Trans_Receive,Supervisory
  Check EM Limits : Subsystem
  Check Engine Limits : Subsystem
  Terminator : Terminator
  HSC_Out : Outport
  wires:
  Bus Creator/1 -> HSC_Out/1  "HSC_Out"
  In1/1 -> Bus Selector/1
  Bus Selector/1 -> Bus Creator/1  "<ESS_Signals_A123>"
  Bus Creator1/1 -> Bus Creator/2  "EM_Messages_Rhinehart"
  Bus Selector/6 -> Check Engine Limits/1(In1)  "<ICE_Torque_Request_Nm>"
  Bus Selector/9 -> Bus Creator/5  "<Trans_Receive>"
  Bus Selector/10 -> Bus Creator/6  "<Supervisory>"
  Bus Creator4/1 -> Bus Creator/4  "Engine_Messages"
  Bus Selector/7 -> Bus Creator4/2  "<Engine_On>"
  Bus Selector/8 -> Bus Creator4/3  "<Engine_Run>"
  Check Engine Limits/1(Out1) -> Bus Creator4/1  "ICE_Torque_Request_Nm"
  Bus Selector/2 -> Check EM Limits/1(EnableReq)  "<Inverter_Enable>"
  Bus Selector/3 -> Check EM Limits/2(In1)  "<Torque_Command>"
  Check EM Limits/2(Torque) -> Bus Creator1/2  "Torque_Command"
  Check EM Limits/1(Enable) -> Bus Creator1/1  "Inverter_Enable"
  Check EM Limits/3(Direction) -> Bus Creator1/3  "Rotation_Direction"
  CAN/1 -> Check EM Limits/3(FromCAN)
  Bus Selector/4 -> Terminator/1  "<Rotation_Direction>"
  Bus Selector/5 -> Bus Creator/3  "<BAS_Infineon_Messages>"
  Clutch/1 -> Check Engine Limits/2(Clutch)

== system EcoSIM3_P2_C2_WIP/Supervisory Controller/PRNDL/Neutral  ==
  Treq : Inport
  CAN : Inport  Port=2
  Enable : EnablePort
  Bus Creator1 : BusCreator  Inputs=6
  Bus Creator2 : BusCreator  Inputs=3
  Bus Creator4 : BusCreator  Inputs=3
  Bus Selector : BusSelector  OutputSignals=ESS_Signals_A123,EM_Messages_Rhinehart.Inverter_Enable,EM_Messages_Rhinehart.Torque_Command,EM_Messages_Rhinehart.Rotation_Direction,BAS_Infineon_Messages,ICE_Request.ICE_Torque_Request_Nm,ICE_Request.Engine_On,ICE_Request.Engine_Run,Trans_Receive,Supervisory
  Check EM Limits : Subsystem
  ICE3 : Constant  Value=0
  ICE6 : Constant  Value=0
  Terminator : Terminator
  Terminator2 : Terminator
  Terminator3 : Terminator
  "HSC_Out " : Outport
  wires:
  Bus Creator1/1 -> "HSC_Out "/1  "HSC_Out"
  Treq/1 -> Bus Selector/1
  Bus Selector/1 -> Bus Creator1/1  "<ESS_Signals_A123>"
  Bus Creator2/1 -> Bus Creator1/2  "EM_Messages_Rhinehart"
  Bus Selector/6 -> Terminator/1  "<ICE_Torque_Request_Nm>"
  Bus Selector/9 -> Bus Creator1/5  "<Trans_Receive>"
  ICE3/1 -> Bus Creator2/2  "Torque_Command"
  Bus Selector/10 -> Bus Creator1/6  "<Supervisory>"
  Bus Creator4/1 -> Bus Creator1/4  "Engine_Messages"
  Bus Selector/7 -> Bus Creator4/2  "<Engine_On>"
  Bus Selector/8 -> Bus Creator4/3  "<Engine_Run>"
  ICE6/1 -> Bus Creator4/1  "ICE_Torque_Request_Nm"
  Bus Selector/2 -> Check EM Limits/1(EnableReq)  "<Inverter_Enable>"
  Bus Selector/3 -> Check EM Limits/2(In1)  "<Torque_Command>"
  Check EM Limits/1(Enable) -> Bus Creator2/1  "Inverter_Enable"
  Check EM Limits/3(Direction) -> Bus Creator2/3
  Check EM Limits/2(Torque) -> Terminator2/1
  CAN/1 -> Check EM Limits/3(FromCAN)
  Bus Selector/4 -> Terminator3/1  "<Rotation_Direction>"
  Bus Selector/5 -> Bus Creator1/3  "<BAS_Infineon_Messages>"

== system EcoSIM3_P2_C2_WIP/Supervisory Controller/PRNDL/Park ==
  Treq : Inport
  CAN : Inport  Port=2
  Enable : EnablePort
  Bus Creator1 : BusCreator  Inputs=6
  Bus Creator2 : BusCreator  Inputs=3
  Bus Creator4 : BusCreator  Inputs=3
  Bus Selector : BusSelector  OutputSignals=ESS_Signals_A123,EM_Messages_Rhinehart,BAS_Infineon_Messages,ICE_Request.ICE_Torque_Request_Nm,ICE_Request.Engine_On,ICE_Request.Engine_Run,Trans_Receive,Supervisory
  Check EM Limits : Subsystem
  ICE1 : Constant  Value=0
  ICE3 : Constant  Value=0
  Terminator2 : Terminator
  Terminator4 : Terminator
  HSC_Out : Outport
  wires:
  Bus Creator1/1 -> HSC_Out/1  "HSC_Out"
  Treq/1 -> Bus Selector/1
  Bus Selector/1 -> Bus Creator1/1  "<ESS_Signals_A123>"
  Bus Creator2/1 -> Bus Creator1/2  "EM_Messages_Rhinehart"
  Bus Selector/4 -> Terminator4/1  "<ICE_Torque_Request_Nm>"
  Bus Selector/7 -> Bus Creator1/5  "<Trans_Receive>"
  Bus Creator4/1 -> Bus Creator1/4  "Engine_Messages"
  Bus Selector/8 -> Bus Creator1/6  "<Supervisory>"
  Bus Selector/5 -> Bus Creator4/2  "<Engine_On>"
  Bus Selector/6 -> Bus Creator4/3  "<Engine_Run>"
  ICE1/1 -> Bus Creator4/1  "ICE_Torque_Request_Nm"
  Bus Selector/2 -> Check EM Limits/1(EM)  "<EM_Messages_Rhinehart>"
  CAN/1 -> Check EM Limits/2(FromCAN)
  Check EM Limits/3(Direction) -> Bus Creator2/3
  Check EM Limits/1(Enable) -> Bus Creator2/1  "Inverter_Enable"
  ICE3/1 -> Bus Creator2/2  "Torque_Command"
  Check EM Limits/2(Torque) -> Terminator2/1
  Bus Selector/3 -> Bus Creator1/3  "<BAS_Infineon_Messages>"

== system EcoSIM3_P2_C2_WIP/Supervisory Controller/PRNDL/Reverse ==
  Treq : Inport
  CAN : Inport  Port=2
  Enable : EnablePort
  Bus Creator : BusCreator  Inputs=6
  Bus Creator1 : BusCreator  Inputs=3
  Bus Creator4 : BusCreator  Inputs=3
  Bus Selector : BusSelector  OutputSignals=ESS_Signals_A123,EM_Messages_Rhinehart.Inverter_Enable,EM_Messages_Rhinehart.Torque_Command,EM_Messages_Rhinehart.Rotation_Direction,BAS_Infineon_Messages,ICE_Request.ICE_Torque_Request_Nm,ICE_Request.Engine_On,ICE_Request.Engine_Run,Trans_Receive,Supervisory
  Check EM Limits : Subsystem
  Ensure Desired Rotation Direction : Subsystem
  Terminator : Terminator
  "HSC_Out " : Outport
  wires:
  Bus Creator/1 -> "HSC_Out "/1  "HSC_Out"
  Treq/1 -> Bus Selector/1
  Bus Selector/1 -> Bus Creator/1  "<ESS_Signals_A123>"
  Bus Selector/3 -> Check EM Limits/3(TorqueReq)  "<Torque_Command>"
  Bus Creator1/1 -> Bus Creator/2  "EM_Messages_Rhinehart"
  Bus Selector/9 -> Bus Creator/5  "<Trans_Receive>"
  Bus Selector/10 -> Bus Creator/6  "<Supervisory>"
  Bus Creator4/1 -> Bus Creator/4  "Engine_Messages"
  Bus Selector/7 -> Bus Creator4/2  "<Engine_On>"
  Bus Selector/8 -> Bus Creator4/3  "<Engine_Run>"
  Bus Selector/6 -> Bus Creator4/1  "<ICE_Torque_Request_Nm>"
  Bus Selector/2 -> Check EM Limits/1(EMEnable)  "<Inverter_Enable>"
  Check EM Limits/1(Enable) -> Bus Creator1/1  "Inverter_Enable"
  Check EM Limits/2(Torque) -> Bus Creator1/2  "Torque_Command"
  Check EM Limits/3(Direction) -> Bus Creator1/3  "Rotation_Direction"
  CAN/1 -> Check EM Limits/2(FromCAN)
  Bus Selector/4 -> Terminator/1  "<Rotation_Direction>"
  Bus Selector/5 -> Bus Creator/3  "<BAS_Infineon_Messages>"

== system EcoSIM3_P2_C2_WIP/Supervisory Controller/Simple Fault Detection/CAN Communication Failures  ==
  In1 : Inport
  Out1 : Outport
  wires:
  In1/1 -> Out1/1

== system EcoSIM3_P2_C2_WIP/Supervisory Controller/Simple Fault Detection/Inverter Temp Selection  ==
  note: This is taking in all of the inverter temperatures and outputing the highest one
  In1 : Inport
  Bus Selector : BusSelector  OutputSignals=M160_Temperature_Set_1.Module_A,M160_Temperature_Set_1.Module_B,M160_Temperature_Set_1.Module_C,M160_Temperature_Set_1.Gate_Driver_Board,M161_Temperature_Set_2.Control_Board_Temperature
  MinMax : MinMax  Function=max
  Mux : Mux  Inputs=5
  Out1 : Outport
  wires:
  In1/1 -> Bus Selector/1
  MinMax/1 -> Out1/1  "Inverter_Temp"
  Bus Selector/4 -> Mux/4  "<Gate_Driver_Board>"
  Bus Selector/5 -> Mux/5  "<Control_Board_Temperature>"
  Bus Selector/3 -> Mux/3  "<Module_C>"
  Bus Selector/1 -> Mux/1  "<Module_A>"
  Bus Selector/2 -> Mux/2  "<Module_B>"
  Mux/1 -> MinMax/1

== system EcoSIM3_P2_C2_WIP/Supervisory Controller/Supervisory_IO/From_Goto ==
  Bus Creator : BusCreator  Inputs=8
  Bus Creator1 : BusCreator  Inputs=1
  Bus Selector1 : BusSelector  OutputSignals=GM_Transmit,ESS_Transmit,EM_Transmit,ICE_Transmit,BAS_Transmit,CP1_Transmit,Mastershift_Transmit
  tag scope: From_Supervisory=global, From_Vehicle=global
  wires:
  Bus Creator/1 -> [From_Vehicle]
  [From_ECUs] -> Bus Selector1/1
  Bus Selector1/2 -> Bus Creator/3  "<ESS_Transmit>"
  Bus Selector1/3 -> Bus Creator/4  "<EM_Transmit>"
  Bus Selector1/4 -> Bus Creator/5  "<ICE_Transmit>"
  Bus Selector1/5 -> Bus Creator/6  "<BAS_Transmit>"
  [From_GCM] -> Bus Creator/1
  [To_Vehicle] -> Bus Creator1/1
  Bus Creator1/1 -> [From_Supervisory]
  Bus Selector1/1 -> Bus Creator/2  "<GM_Transmit>"
  Bus Selector1/6 -> Bus Creator/7  "<CP1_Transmit>"
  Bus Selector1/7 -> Bus Creator/8  "<Mastershift_Transmit>"

== system EcoSIM3_P2_C2_WIP/Supervisory Controller/Supervisory_IO/VNT Kvaser ==
  CAN Rx : Subsystem
  CAN Tx : Subsystem
  Electrical Rx : Subsystem
  Electrical Tx : Subsystem
  Spine : Subsystem
  wires:
  Electrical Rx/1(Electrical_Rx) -> Spine/1(Electrical Rx)
  CAN Rx/1(CAN_Rx) -> Spine/2(CAN Rx)
  Spine/1(ElectricalTx) -> Electrical Tx/1(Electrical Tx)
  Spine/2(CANTx) -> CAN Tx/1(CAN Tx)

== system EcoSIM3_P2_C2_WIP/Supervisory Controller/Supervisory_IO/VNT Vector ==
  CAN Rx : Subsystem
  CAN Tx : Subsystem
  Electrical Rx : Subsystem
  Electrical Tx : Subsystem
  Spine : Subsystem
  wires:
  Electrical Rx/1(Electrical_Rx) -> Spine/1(Electrical Rx)
  CAN Rx/1(CAN_Rx) -> Spine/2(CAN Rx)
  Spine/1(ElectricalTx) -> Electrical Tx/1(Electrical Tx)
  Spine/2(CANTx) -> CAN Tx/1(CAN Tx)

== system EcoSIM3_P2_C2_WIP/Driver/PI Controller/Dyno Data Variant/AcclnTest250 ==
  CycleTime : Constant  Value=AcclnTest250.time(end)
  From Workspace : FromWorkspace  VariableName=[AcclnTest250.time',AcclnTest250.Alpha_percent']  SampleTime=0
  From Workspace1 : FromWorkspace  VariableName=[AcclnTest250.time',AcclnTest250.Brake_percent']  SampleTime=0
  From Workspace10 : FromWorkspace  VariableName=[AcclnTest250.time',AcclnTest250.bcm_soc']  SampleTime=0
  From Workspace11 : FromWorkspace  VariableName=[AcclnTest250.time',AcclnTest250.bcm_cell_tmax']  SampleTime=0
  From Workspace12 : FromWorkspace  VariableName=[AcclnTest250.time',AcclnTest250.bcm_cell_tmin']  SampleTime=0
  From Workspace2 : FromWorkspace  VariableName=[AcclnTest250.time',AcclnTest250.Speed_m_per_s']  SampleTime=0
  From Workspace3 : FromWorkspace  VariableName=[AcclnTest250.time',AcclnTest250.Driver_Req_Trq']  SampleTime=0
  From Workspace4 : FromWorkspace  VariableName=[AcclnTest250.time',AcclnTest250.bcm_ibat']  SampleTime=0
  From Workspace5 : FromWorkspace  VariableName=[AcclnTest250.time',AcclnTest250.bcm_vbat']  SampleTime=0
  From Workspace6 : FromWorkspace  VariableName=[AcclnTest250.time',AcclnTest250.D1_Commanded_Trq']  SampleTime=0
  From Workspace7 : FromWorkspace  VariableName=[AcclnTest250.time',AcclnTest250.EM_Trq_Cmd']  SampleTime=0
  From Workspace8 : FromWorkspace  VariableName=[AcclnTest250.time',AcclnTest250.Motor_Speed']  SampleTime=0
  From Workspace9 : FromWorkspace  VariableName=[AcclnTest250.time',AcclnTest250.D2_Trq_Feedback']  SampleTime=0
  Gain : Gain
  Gain1 : Gain
  Terminator{,1..12} (13 alike) : Terminator
  n : Gain  Gain=-1
  n1 : Gain  Gain=-1
  rpmtoradps : Gain  Gain=-0.1047
  Alpha : Outport
  Beta : Outport  Port=2
  tag scope: CycleTime=global, DynoCellTMax=global, DynoCellTMin=global, DynoSpeed=global
  wires:
  From Workspace/1 -> Gain1/1, Alpha/1
  From Workspace1/1 -> Gain/1, Beta/1
  From Workspace2/1 -> [DynoSpeed], Terminator/1  "Dyno_Speed"
  From Workspace3/1 -> Terminator1/1  "Dyno_Drv_Trq_Req"
  From Workspace4/1 -> n1/1
  From Workspace5/1 -> Terminator3/1  "Dyno_bcm_vbat"
  From Workspace6/1 -> Terminator4/1  "Dyno_D1_Cmdd_Trq"
  From Workspace7/1 -> Terminator5/1  "Dyno_EM_Trq_Cmd"
  rpmtoradps/1 -> Terminator6/1  "Dyno_MotorSpd_radpers"
  From Workspace8/1 -> rpmtoradps/1  "Dyno_MotorSpd_rpm"
  n/1 -> Terminator7/1  "Dyno_D2_Trq_Fdbk"
  From Workspace9/1 -> n/1
  CycleTime/1 -> [CycleTime]
  Gain/1 -> Terminator8/1  "Dyno_Brk_Pct"
  n1/1 -> Terminator2/1  "Dyno_bcm_ibat"
  From Workspace10/1 -> Terminator9/1  "Dyno_bcm_soc"
  Gain1/1 -> Terminator10/1  "Dyno_Alpha"
  From Workspace11/1 -> [DynoCellTMax], Terminator11/1  "Dyno_bcm_cell_tmax"
  From Workspace12/1 -> [DynoCellTMin], Terminator12/1  "Dyno_bcm_cell_tmin"
